simulink model "gm_two_stage_hdl_coder"  (R2021b)
settings: Solver=VariableStepAuto  StartTime=0.0  StopTime=3  RelTol=1e-3
undefined symbols (not defined in the file or in its folder): fsample, taps1, taps2
libraries: simulink x1
settings Model: Creator=pablo  LastModifiedBy=pablo
settings SolverCC: AutoInsertRateTranBlk=on
settings OptimizationCC: BlockReduction=off  ConditionallyExecuteInputs=off
settings DebuggingCC: InheritedTsInSrcMsg=none  SingleTaskRateTransMsg=error

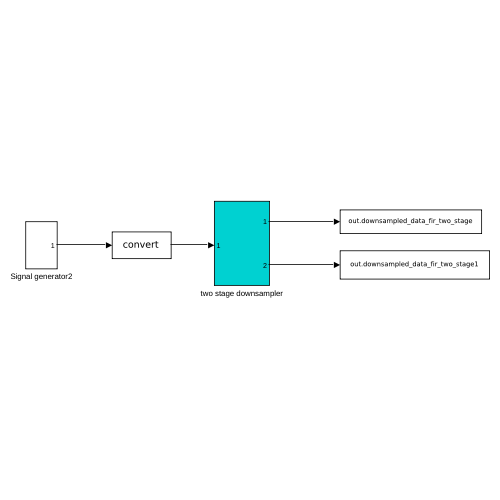
[thumbnail: Simulink's stored preview of the top-level diagram]
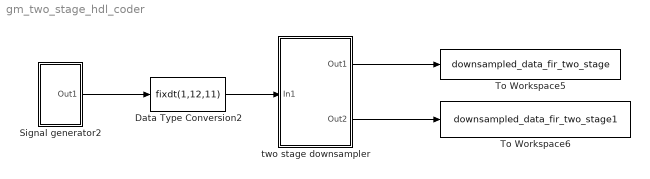
== system gm_two_stage_hdl_coder ==
  Data Type Conversion2 : DataTypeConversion  OutDataTypeStr=fixdt(1,12,11)
  Signal generator2 : Subsystem
  To Workspace5 : ToWorkspace  VariableName=downsampled_data_fir_two_stage  SampleTime=-1
  To Workspace6 : ToWorkspace  VariableName=downsampled_data_fir_two_stage1  SampleTime=-1
  two stage downsampler : Subsystem
  wires:
  two stage downsampler/2(Out2) -> To Workspace6/1
  two stage downsampler/1(Out1) -> To Workspace5/1
  Data Type Conversion2/1 -> two stage downsampler/1(In1)
  Signal generator2/1(Out1) -> Data Type Conversion2/1

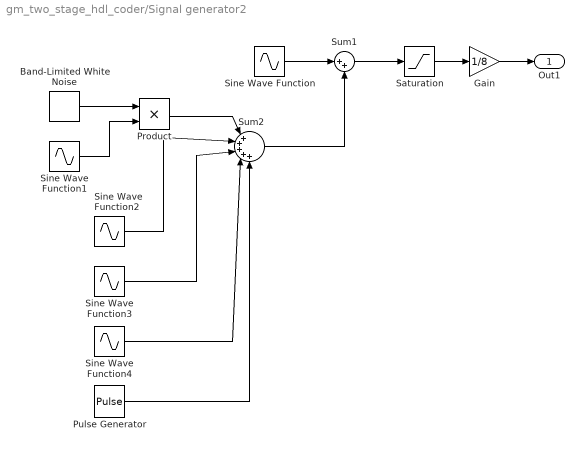
== system gm_two_stage_hdl_coder/Signal generator2 ==
  Band-Limited White Noise : simulink/Sources/Band-Limited White Noise  Cov=[0.00001]  Ts=1/fsample  seed=[25]
  Gain : Gain  Gain=1/8
  Product : Product
  Pulse Generator : DiscretePulseGenerator  Amplitude=0.8  Period=24  PulseWidth=12  SampleTime=1/fsample
  Saturation : Saturate  UpperLimit=8  LowerLimit=-8
  Sine Wave Function : Sin  SineType=Sample based  Frequency=50*2*pi  Samples=fsample/50  SampleTime=1/fsample
  Sine Wave Function1 : Sin  Frequency=200*2*pi  Samples=fsample/50  SampleTime=1/fsample
  Sine Wave Function2 : Sin  Amplitude=0.3  Frequency=3100*2*pi  Phase=3  Samples=fsample/50  SampleTime=1/fsample
  Sine Wave Function3 : Sin  Amplitude=0.5  Frequency=2500*2*pi  Samples=fsample/50  SampleTime=1/fsample
  Sine Wave Function4 : Sin  Amplitude=0.5  Frequency=5000*2*pi  Samples=fsample/50  SampleTime=1/fsample
  Sum1 : Sum  Inputs=|++
  Sum2 : Sum  Inputs=|+++++
  Out1 : Outport
  wires:
  Gain/1 -> Out1/1
  Saturation/1 -> Gain/1
  Sum1/1 -> Saturation/1
  Sum2/1 -> Sum1/2
  Pulse Generator/1 -> Sum2/5
  Product/1 -> Sum2/1
  Band-Limited White Noise/1 -> Product/1
  Sine Wave Function1/1 -> Product/2
  Sine Wave Function4/1 -> Sum2/4
  Sine Wave Function/1 -> Sum1/1
  Sine Wave Function3/1 -> Sum2/3
  Sine Wave Function2/1 -> Sum2/2

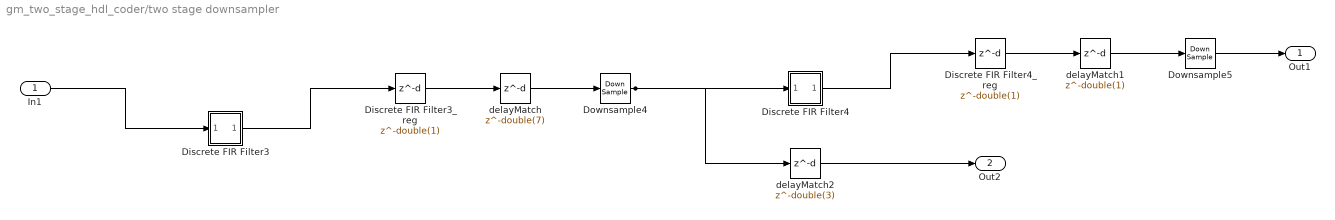
== system gm_two_stage_hdl_coder/two stage downsampler ==
  In1 : Inport  OutDataTypeStr=fixdt(1, 12, 11)  PortDimensions=1  SampleTime=1e-05
  Discrete FIR Filter3 : Subsystem
  Discrete FIR Filter3_reg : Delay  DelayLength=double(1)  InitialCondition=0  SampleTime=1e-05
  Discrete FIR Filter4 : Subsystem
  Discrete FIR Filter4_reg : Delay  DelayLength=double(1)  InitialCondition=0  SampleTime=9e-05
  Downsample4 : DownSample  N=double(9)  phase=double(0)  RateOptions=Allow multirate processing
  Downsample5 : DownSample  N=double(4)  phase=double(0)  RateOptions=Allow multirate processing
  delayMatch : Delay  DelayLength=double(7)  InitialCondition=0  SampleTime=1e-05
  delayMatch1 : Delay  DelayLength=double(1)  InitialCondition=0  SampleTime=9e-05
  delayMatch2 : Delay  DelayLength=double(3)  InitialCondition=0  SampleTime=9e-05
  Out1 : Outport  SampleTime=0.00036
  Out2 : Outport  Port=2  SampleTime=9e-05
  wires:
  In1/1 -> Discrete FIR Filter3/1(In1)
  delayMatch/1 -> Downsample4/1
  delayMatch1/1 -> Downsample5/1
  delayMatch2/1 -> Out2/1
  Downsample5/1 -> Out1/1
  Discrete FIR Filter3/1(Out1) -> Discrete FIR Filter3_reg/1
  Discrete FIR Filter4/1(Out1) -> Discrete FIR Filter4_reg/1
  Discrete FIR Filter3_reg/1 -> delayMatch/1
  Discrete FIR Filter4_reg/1 -> delayMatch1/1
  Downsample4/1 -> delayMatch2/1, Discrete FIR Filter4/1(In1)

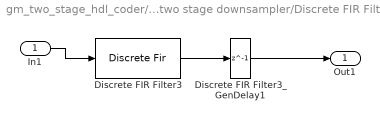
== system gm_two_stage_hdl_coder/two stage downsampler/Discrete FIR Filter3 ==
  In1 : Inport
  Discrete FIR Filter3 : DiscreteFir  Coefficients=taps1  InputProcessing=Columns as channels (frame based)  SampleTime=1/fsample  CoefDataTypeStr=fixdt(1,16,15)  OutDataTypeStr=Inherit: Same as input
  Discrete FIR Filter3_GenDelay1 : Delay  DelayLength=1
  Out1 : Outport
  wires:
  In1/1 -> Discrete FIR Filter3/1
  Discrete FIR Filter3/1 -> Discrete FIR Filter3_GenDelay1/1
  Discrete FIR Filter3_GenDelay1/1 -> Out1/1

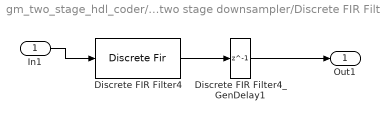
== system gm_two_stage_hdl_coder/two stage downsampler/Discrete FIR Filter4 ==
  In1 : Inport
  Discrete FIR Filter4 : DiscreteFir  Coefficients=taps2  InputProcessing=Columns as channels (frame based)  CoefDataTypeStr=fixdt(1,16,15)  OutDataTypeStr=Inherit: Same as input
  Discrete FIR Filter4_GenDelay1 : Delay  DelayLength=1
  Out1 : Outport
  wires:
  In1/1 -> Discrete FIR Filter4/1
  Discrete FIR Filter4/1 -> Discrete FIR Filter4_GenDelay1/1
  Discrete FIR Filter4_GenDelay1/1 -> Out1/1
